simulink model "Inv_Pend_Sim_Compressed"  (R2018a)
settings: Solver=FixedStepAuto  StartTime=0.0  StopTime=15  FixedStep=0.002  RelTol=1e-3
values from neighbouring files (symbols this model uses):
  Ad = sysd.A    [Project_Paper_Optimizer.m]
  b_0 = x(1,7)    [INV_PEND_ADRC_PSO.m]    (also in Project_Paper_Optimizer.m = m_pop(i,7))
  Bd = sysd.B    [Project_Paper_Optimizer.m]
  beta_01c = m_pop(i,9)    [Project_Paper_Optimizer.m]
  beta_01p = m_pop(i,8)    [Project_Paper_Optimizer.m]
  beta_02c = m_pop(i,11)    [Project_Paper_Optimizer.m]
  beta_02p = m_pop(i,10)    [Project_Paper_Optimizer.m]
  beta_03c = m_pop(i,13)    [Project_Paper_Optimizer.m]
  beta_03p = m_pop(i,12)    [Project_Paper_Optimizer.m]
  c_c = m_pop(i,6)    [Project_Paper_Optimizer.m]
  c_p = m_pop(i,5)    [Project_Paper_Optimizer.m]
  Cd = sysd.C    [Project_Paper_Optimizer.m]
  d_p = 0.0127    [INV_PEND_ADRC_PSO.m]    (also in Project_Paper_Optimizer.m)
  h = 0.001    [INV_PEND_ADRC_PSO.m]    (also in NSDE_2.m = 1 - (m_pop(:,1)./g).^2; Project_Paper_Optimizer.m = 0.002; RPD_NSGA_2.m = 1 - sqrt(m_pop(:,1)./g))
  h_1c = m_pop(i,2)    [Project_Paper_Optimizer.m]
  h_1p = m_pop(i,1)    [Project_Paper_Optimizer.m]
  r_c = m_pop(i,4)    [Project_Paper_Optimizer.m]
  r_p = m_pop(i,3)    [Project_Paper_Optimizer.m]
  Ts = 0.002    [Project_Paper_Optimizer.m]
undefined symbols (not defined in the file or in its folder): sigbuilder_block
settings Model: Creator=pc01  LastModifiedBy=pc01

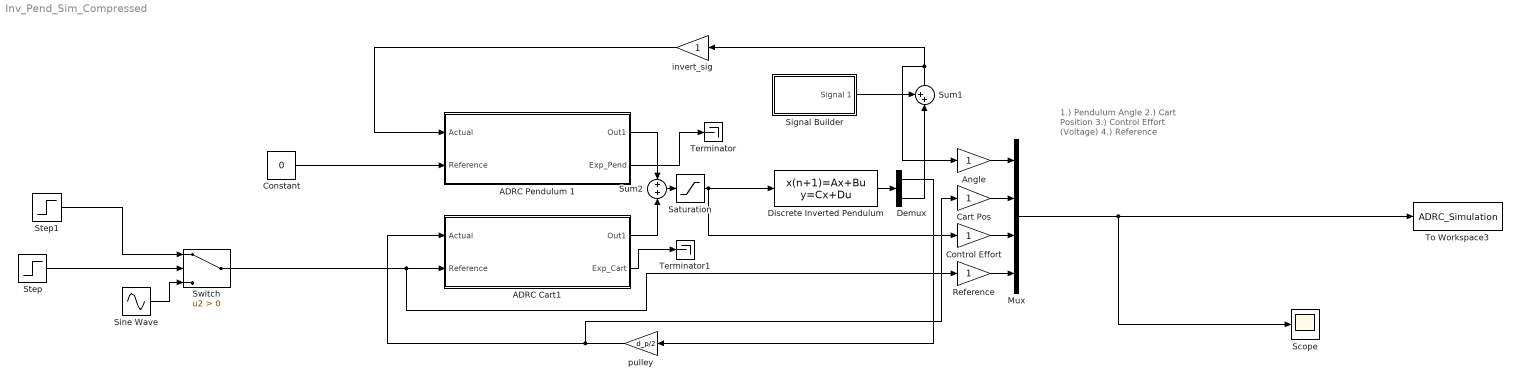
== system Inv_Pend_Sim_Compressed ==
  note: 1.) Pendulum Angle
      | 2.) Cart Position
      | 3.) Control Effort (Voltage)
      | 4.) Reference
  ADRC Cart1 : Subsystem
  ADRC Pendulum 1 : Subsystem
  Angle : Gain
  "Cart Pos " : Gain
  Constant : Constant  Value=0  SampleTime=Ts
  Control Effort : Gain
  Demux : Demux  Outputs=2
  Discrete Inverted Pendulum : DiscreteStateSpace  A=Ad  B=Bd  C=Cd  D=[0;0]  InitialCondition=[0 0 0 0]  SampleTime=Ts
  Mux : Mux
  Reference : Gain
  Saturation : Saturate  UpperLimit=25  LowerLimit=-25
  Scope : Scope
  Signal Builder : Subsystem  Tag=STV Subsys  LoadFcn=sigbuilder_block('load');  StartFcn=sigbuilder_block('start');  StopFcn=sigbuilder_block('stop');  ClipboardFcn=sigbuilder_block('clipboard');  mask(Sigbuilder block){tuvar=[0:10]}
      mask help: Simulink:masks:SigbuilderBlock_MD
      mask init:
      | if ~strcmp(get_param(bdroot(gcbh),'SimulationStatus'),'stopped') tuvar = sigbuilder_block('maskInit'); end
      settings: CopyFcn=sigbuilder_block('copy');  DeleteFcn=sigbuilder_block('delete');  ModelCloseFcn=sigbuilder_block('modelClose');  PreSaveFcn=sigbuilder_block('preSave');  PauseFcn=sigbuilder_block('pause');  ContinueFcn=sigbuilder_block('continue');  NameChangeFcn=sigbuilder_block('namechange');  OpenFcn=sigbuilder_block('open',[437.6 199.2 550.4 400 ]);  CloseFcn=sigbuilder_block('close');
      mask Display: plot(0, 0, 100, 100,[2, 2, 32, 32, 2], [68, 8, 8, 68, 68],[32, 2], [38, 38], [32, 19, 2],[53, 60, 44], [32, 17, 17, 2],[16, 16, 31, 31]);txt = getActiveGroup(gcbh);text(2, 100, txt,'verticalAlignment', 'top');
  Sine Wave : Sin  Amplitude=0.1  SampleTime=Ts
  Step : Step  Time=8  Before=1  After=0  SampleTime=Ts
  Step1 : Step  Time=0.5  After=0.1  SampleTime=Ts
  Sum1 : Sum  Inputs=++|
  Sum2 : Sum  Inputs=+|+
  Switch : Switch  Criteria=u2 > Threshold
  Terminator : Terminator
  Terminator1 : Terminator
  To Workspace3 : ToWorkspace  VariableName=ADRC_Simulation  SaveFormat=Timeseries  SampleTime=-1
  invert_sig : Gain
  "pulley " : Gain  Gain=d_p/2
  wires:
  Sine Wave/1 -> Switch/3
  Demux/1 -> "pulley "/1
  ADRC Cart1/1(Out1) -> Sum2/2
  "pulley "/1 -> "Cart Pos "/1, ADRC Cart1/1(Actual)
  Saturation/1 -> Discrete Inverted Pendulum/1, Control Effort/1
  Discrete Inverted Pendulum/1 -> Demux/1
  ADRC Pendulum 1/1(Out1) -> Sum2/1
  Step/1 -> Switch/2
  Angle/1 -> Mux/1
  invert_sig/1 -> ADRC Pendulum 1/1(Actual)
  ADRC Cart1/2(Exp_Cart) -> Terminator1/1
  "Cart Pos "/1 -> Mux/2
  Switch/1 -> Reference/1, ADRC Cart1/2(Reference)
  Demux/2 -> Sum1/2
  Sum1/1 -> Angle/1, invert_sig/1
  Step1/1 -> Switch/1
  Reference/1 -> Mux/4
  ADRC Pendulum 1/2(Exp_Pend) -> Terminator/1
  Mux/1 -> Scope/1, To Workspace3/1
  Constant/1 -> ADRC Pendulum 1/2(Reference)
  Signal Builder/1(Signal 1) -> Sum1/1
  Sum2/1 -> Saturation/1
  Control Effort/1 -> Mux/3

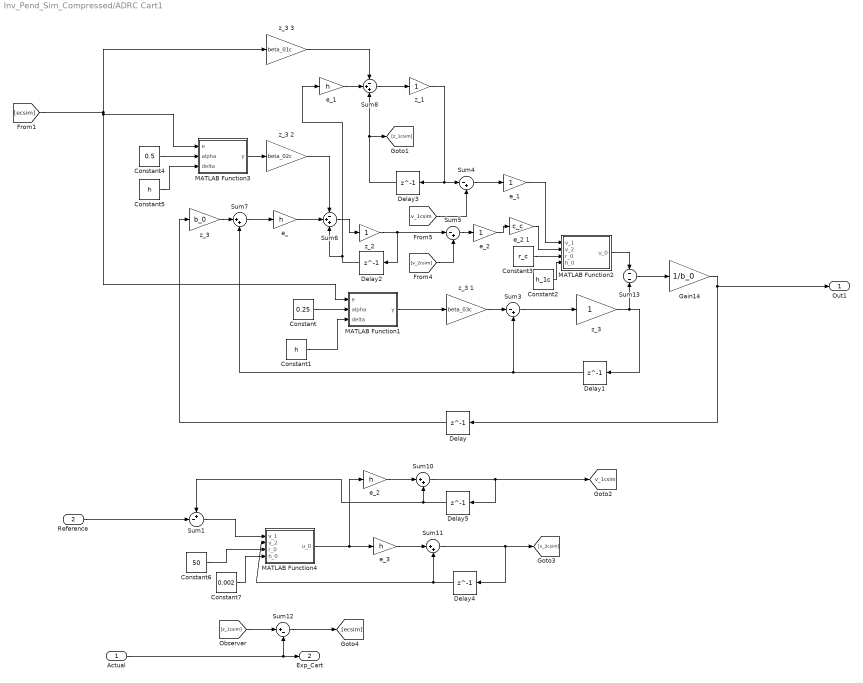
== system Inv_Pend_Sim_Compressed/ADRC Cart1 ==
  Actual : Inport
  Reference : Inport  Port=2
  Constant : Constant  Value=0.25
  Constant1 : Constant  Value=h
  Constant2 : Constant  Value=h_1c
  Constant3 : Constant  Value=r_c
  Constant4 : Constant  Value=0.5
  Constant5 : Constant  Value=h
  Constant6 : Constant  Value=50
  Constant7 : Constant  Value=0.002
  Delay{,1..5} (6 alike) : Delay  DelayLength=1  InitialCondition=0  SampleTime=Ts
  Gain14 : Gain  Gain=1/b_0
  MATLAB Function1 : MATLAB Function  TreatAsAtomicUnit=on
  MATLAB Function2 : MATLAB Function  TreatAsAtomicUnit=on
  MATLAB Function3 : MATLAB Function  TreatAsAtomicUnit=on
  MATLAB Function4 : MATLAB Function  TreatAsAtomicUnit=on
  Sum1 : Sum  Inputs=+-|
  Sum10 : Sum  Inputs=|++
  Sum11 : Sum  Inputs=|++
  Sum12 : Sum  Inputs=|+-
  Sum13 : Sum  Inputs=-|-
  Sum3 : Sum  Inputs=|-+
  Sum4 : Sum  Inputs=|-+
  Sum5 : Sum  Inputs=|-+
  Sum6 : Sum  Inputs=-++
  Sum7 : Sum  Inputs=|++
  Sum8 : Sum  Inputs=-++
  e_{,1..3} (4 alike) : Gain  Gain=h
  "e_1 " : Gain
  "e_2 " : Gain
  e_2 1 : Gain  Gain=c_c
  z_1 : Gain
  z_2 : Gain
  z_3 : Gain  Gain=b_0
  "z_3 " : Gain
  z_3 1 : Gain  Gain=beta_03c
  z_3 2 : Gain  Gain=beta_02c
  z_3 3 : Gain  Gain=beta_01c
  Out1 : Outport
  Exp_Cart : Outport  Port=2
  tag scope: v_1csim=global
  wires:
  Delay4/1 -> MATLAB Function4/2(v_2), Sum11/2
  Delay2/1 -> e_1/1, Sum6/3
  [z_1csim] -> Sum12/1
  Sum5/1 -> "e_2 "/1
  z_3 3/1 -> Sum8/1
  Sum7/1 -> e_/1
  Sum13/1 -> Gain14/1
  z_1/1 -> Delay3/1, Sum4/1
  Delay1/1 -> Sum3/2, Sum7/2
  [ecsim] -> MATLAB Function1/1(e), MATLAB Function3/1(e), z_3 3/1
  Constant3/1 -> MATLAB Function2/3(r_0)
  z_2/1 -> Delay2/1, Sum5/1
  [v_2csim] -> Sum5/2
  [v_1csim] -> Sum4/2
  Constant/1 -> MATLAB Function1/2(alpha)
  e_1/1 -> Sum8/2
  MATLAB Function2/1(u_0) -> Sum13/1
  Sum11/1 -> Delay4/1, [v_2csim]
  Sum3/1 -> "z_3 "/1
  e_3/1 -> Sum11/1
  Constant6/1 -> MATLAB Function4/3(r_0)
  Delay3/1 -> [z_1csim], Sum8/3
  Constant1/1 -> MATLAB Function1/3(delta)
  e_/1 -> Sum6/2
  Delay5/1 -> Sum10/2, Sum1/1
  Constant7/1 -> MATLAB Function4/4(h_0)
  e_2/1 -> Sum10/1
  Constant2/1 -> MATLAB Function2/4(h_0)
  "z_3 "/1 -> Delay1/1, Sum13/2
  Gain14/1 -> Out1/1, Delay/1
  Sum6/1 -> z_2/1
  z_3/1 -> Sum7/1
  z_3 1/1 -> Sum3/1
  Constant4/1 -> MATLAB Function3/2(alpha)
  z_3 2/1 -> Sum6/1
  Constant5/1 -> MATLAB Function3/3(delta)
  Sum4/1 -> "e_1 "/1
  e_2 1/1 -> MATLAB Function2/2(v_2)
  "e_1 "/1 -> MATLAB Function2/1(v_1)
  Sum8/1 -> z_1/1
  Delay/1 -> z_3/1
  Actual/1 -> Exp_Cart/1, Sum12/2
  "e_2 "/1 -> e_2 1/1
  Sum1/1 -> MATLAB Function4/1(v_1)
  MATLAB Function4/1(u_0) -> e_2/1, e_3/1
  Sum10/1 -> [v_1csim], Delay5/1
  Reference/1 -> Sum1/2
  Sum12/1 -> [ecsim]
  MATLAB Function3/1(y) -> z_3 2/1
  MATLAB Function1/1(y) -> z_3 1/1

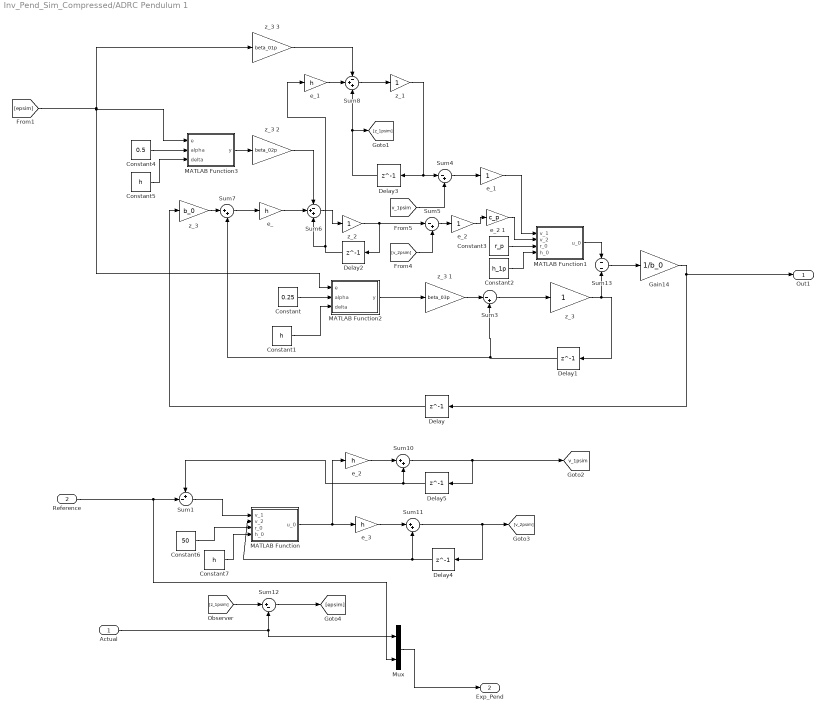
== system Inv_Pend_Sim_Compressed/ADRC Pendulum 1 ==
  Actual : Inport
  Reference : Inport  Port=2
  Constant : Constant  Value=0.25
  Constant1 : Constant  Value=h
  Constant2 : Constant  Value=h_1p
  Constant3 : Constant  Value=r_p
  Constant4 : Constant  Value=0.5
  Constant5 : Constant  Value=h
  Constant6 : Constant  Value=50
  Constant7 : Constant  Value=h
  Delay{,1..5} (6 alike) : Delay  DelayLength=1  InitialCondition=0  SampleTime=Ts
  Gain14 : Gain  Gain=1/b_0
  MATLAB Function : MATLAB Function  TreatAsAtomicUnit=on
  MATLAB Function1 : MATLAB Function  TreatAsAtomicUnit=on
  MATLAB Function2 : MATLAB Function  TreatAsAtomicUnit=on
  MATLAB Function3 : MATLAB Function  TreatAsAtomicUnit=on
  Mux : Mux  Inputs=2
  Sum1 : Sum  Inputs=+-|
  Sum10 : Sum  Inputs=|++
  Sum11 : Sum  Inputs=|++
  Sum12 : Sum  Inputs=|+-
  Sum13 : Sum  Inputs=-|-
  Sum3 : Sum  Inputs=|-+
  Sum4 : Sum  Inputs=|-+
  Sum5 : Sum  Inputs=|-+
  Sum6 : Sum  Inputs=-++
  Sum7 : Sum  Inputs=|++
  Sum8 : Sum  Inputs=-++
  e_{,1..3} (4 alike) : Gain  Gain=h
  "e_1 " : Gain
  "e_2 " : Gain
  e_2 1 : Gain  Gain=c_p
  z_1 : Gain
  z_2 : Gain
  z_3 : Gain  Gain=b_0
  "z_3 " : Gain
  z_3 1 : Gain  Gain=beta_03p
  z_3 2 : Gain  Gain=beta_02p
  z_3 3 : Gain  Gain=beta_01p
  Out1 : Outport
  Exp_Pend : Outport  Port=2
  tag scope: v_1psim=global
  wires:
  Delay4/1 -> MATLAB Function/2(v_2), Sum11/2
  Delay2/1 -> e_1/1, Sum6/3
  [z_1psim] -> Sum12/1
  Sum5/1 -> "e_2 "/1
  Actual/1 -> Mux/1, Sum12/2
  z_3 3/1 -> Sum8/1
  Sum7/1 -> e_/1
  Sum13/1 -> Gain14/1
  z_1/1 -> Delay3/1, Sum4/1
  Delay1/1 -> Sum3/2, Sum7/2
  [epsim] -> MATLAB Function2/1(e), MATLAB Function3/1(e), z_3 3/1
  Constant3/1 -> MATLAB Function1/3(r_0)
  z_2/1 -> Delay2/1, Sum5/1
  [v_2psim] -> Sum5/2
  [v_1psim] -> Sum4/2
  Constant/1 -> MATLAB Function2/2(alpha)
  e_1/1 -> Sum8/2
  MATLAB Function1/1(u_0) -> Sum13/1
  Sum11/1 -> Delay4/1, [v_2psim]
  Sum3/1 -> "z_3 "/1
  e_3/1 -> Sum11/1
  Constant6/1 -> MATLAB Function/3(r_0)
  Delay3/1 -> [z_1psim], Sum8/3
  Constant1/1 -> MATLAB Function2/3(delta)
  e_/1 -> Sum6/2
  Delay5/1 -> Sum10/2, Sum1/1
  Constant7/1 -> MATLAB Function/4(h_0)
  e_2/1 -> Sum10/1
  Constant2/1 -> MATLAB Function1/4(h_0)
  "z_3 "/1 -> Delay1/1, Sum13/2
  Gain14/1 -> Out1/1, Delay/1
  Sum6/1 -> z_2/1
  z_3/1 -> Sum7/1
  z_3 1/1 -> Sum3/1
  Constant4/1 -> MATLAB Function3/2(alpha)
  z_3 2/1 -> Sum6/1
  Constant5/1 -> MATLAB Function3/3(delta)
  Sum4/1 -> "e_1 "/1
  e_2 1/1 -> MATLAB Function1/2(v_2)
  "e_1 "/1 -> MATLAB Function1/1(v_1)
  Sum8/1 -> z_1/1
  Delay/1 -> z_3/1
  Mux/1 -> Exp_Pend/1
  "e_2 "/1 -> e_2 1/1
  Sum1/1 -> MATLAB Function/1(v_1)
  MATLAB Function/1(u_0) -> e_2/1, e_3/1
  Sum10/1 -> [v_1psim], Delay5/1
  Reference/1 -> Sum1/2, Mux/2
  Sum12/1 -> [epsim]
  MATLAB Function3/1(y) -> z_3 2/1
  MATLAB Function2/1(y) -> z_3 1/1

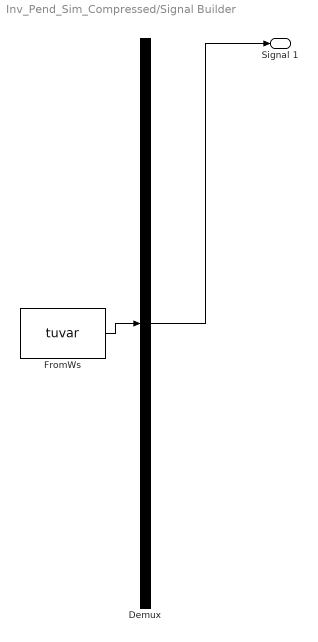
== system Inv_Pend_Sim_Compressed/Signal Builder ==
  Demux : Demux  Tag=STV Demux  Outputs=1
  FromWs : FromWorkspace  Tag=STV FromWs  VariableName=tuvar  SampleTime=Ts
      SigBuilderData=|
      | common.afterFinalStr = 'Extrapolate'
      | common.sampleTime = 'Ts'
      | dataSet.timeRange = [0 10]
      | dataSet.name = 'Group 1'
      | sbobj.Groups.Name = 'Group 1'
      | sbobj.Groups.Signals.Name = 'Signal 1'
      | sbobj.Groups.Signals.XData = [0 5.5 5.5 5.52 5.52 10]
      | sbobj.Groups.Signals.YData = [0 0 0.087 0.087 0 0]
  Signal 1 : Outport  Tag=STV Outport
  wires:
  Demux/1 -> Signal 1/1
  FromWs/1 -> Demux/1

== matlab function Inv_Pend_Sim_Compressed/ADRC Cart1/MATLAB Function3 ==
  data: e input; y output; alpha input; delta input
function y = fal(e, alpha, delta)

    if (abs(e) <= delta)
        fal1 = e/(delta^(1-alpha));
    else
        fal1 = (abs(e)^alpha)*sign(e);
    end
    
y = fal1;

== matlab function Inv_Pend_Sim_Compressed/ADRC Cart1/MATLAB Function1 ==
  data: e input; y output; alpha input; delta input
function y = fal(e, alpha, delta)

    if (abs(e) <= delta)
        fal1 = e/(delta^(1-alpha));
    else
        fal1 = (abs(e)^alpha)*sign(e);
    end
    
y = fal1;

== matlab function Inv_Pend_Sim_Compressed/ADRC Cart1/MATLAB Function2 ==
  data: v_1 input; u_0 output; v_2 input; r_0 input; h_0 input
function u_0 = fhan(v_1, v_2, r_0, h_0)
   

    d = h_0*(r_0)^2;
    a_0 = h_0*v_2;
    y = v_1+a_0;
    a_1 = sqrt(d*(d+8*abs(y)));
    a_2 = a_0+(sign(y)*(a_1 - d))/2;
    s_y = (sign(y + d) - sign(y - d))/2;
    a = (a_0 + y - a_2)*s_y + a_2;
    s_a = (sign(a + d) - sign(a - d))/2;
    fhan_ = -r_0*(((a/d)-sign(a))*s_a)-(r_0*sign(a));

    u_0 = fhan_;
end

== matlab function Inv_Pend_Sim_Compressed/ADRC Cart1/MATLAB Function4 ==
  data: v_1 input; u_0 output; v_2 input; r_0 input; h_0 input
function u_0 = fhan(v_1, v_2, r_0, h_0)
   

    d = h_0*(r_0)^2;
    a_0 = h_0*v_2;
    y = v_1+a_0;
    a_1 = sqrt(d*(d+8*abs(y)));
    a_2 = a_0+(sign(y)*(a_1 - d))/2;
    s_y = (sign(y + d) - sign(y - d))/2;
    a = (a_0 + y - a_2)*s_y + a_2;
    s_a = (sign(a + d) - sign(a - d))/2;
    fhan_ = -r_0*(((a/d)-sign(a))*s_a)-(r_0*sign(a));

    u_0 = fhan_;
end

== matlab function Inv_Pend_Sim_Compressed/ADRC Pendulum 1/MATLAB Function ==
  data: v_1 input; u_0 output; v_2 input; r_0 input; h_0 input
function u_0 = fhan(v_1, v_2, r_0, h_0)
   

    d = h_0*(r_0)^2;
    a_0 = h_0*v_2;
    y = v_1+a_0;
    a_1 = sqrt(d*(d+8*abs(y)));
    a_2 = a_0+(sign(y)*(a_1 - d))/2;
    s_y = (sign(y + d) - sign(y - d))/2;
    a = (a_0 + y - a_2)*s_y + a_2;
    s_a = (sign(a + d) - sign(a - d))/2;
    u_0 = -r_0*(((a/d)-sign(a))*s_a)-(r_0*sign(a));

end

== matlab function Inv_Pend_Sim_Compressed/ADRC Pendulum 1/MATLAB Function1 ==
  data: v_1 input; u_0 output; v_2 input; r_0 input; h_0 input
function u_0 = fhan(v_1, v_2, r_0, h_0)
   

    d = h_0*(r_0)^2;
    a_0 = h_0*v_2;
    y = v_1+a_0;
    a_1 = sqrt(d*(d+8*abs(y)));
    a_2 = a_0+(sign(y)*(a_1 - d))/2;
    s_y = (sign(y + d) - sign(y - d))/2;
    a = (a_0 + y - a_2)*s_y + a_2;
    s_a = (sign(a + d) - sign(a - d))/2;
    fhan_ = -r_0*(((a/d)-sign(a))*s_a)-(r_0*sign(a));

    u_0 = fhan_;
end

== matlab function Inv_Pend_Sim_Compressed/ADRC Pendulum 1/MATLAB Function2 ==
  data: e input; y output; alpha input; delta input
function y = fal(e, alpha, delta)

    if (abs(e) <= delta)
        fal1 = e/(delta^(1-alpha));
    else
        fal1 = (abs(e)^alpha)*sign(e);
    end
    
    y = fal1;
end

== matlab function Inv_Pend_Sim_Compressed/ADRC Pendulum 1/MATLAB Function3 ==
  data: e input; y output; alpha input; delta input
function y = fal(e, alpha, delta)

    if (abs(e) <= delta)
        fal1 = e/(delta^(1-alpha));
    else
        fal1 = (abs(e)^alpha)*sign(e);
    end
    
y = fal1;
